simulink model "Ydq_noise_model"  (R2021b)
settings: Solver=FixedStepAuto  StartTime=0.0  StopTime=t_end  FixedStep=1e-5  RelTol=1e-3
undefined symbols (not defined in the file or in its folder): base, omega0, V0, V_p
libraries: spsControlledVoltageSourceLib x3, simulink x2, spsGroundLib x2, spsabctodq0Lib x1, spsdq0toabcLib x1, spsThreePhaseVIMeasurementLib x1, spspowerguiLib x1
settings Model: Creator=lpwoolcock  LastModifiedBy=lpwoolcock
settings SolverCC: AlgebraicLoopSolver=TrustRegion
settings DebuggingCC: SFMachineParentedDataDiag=warning

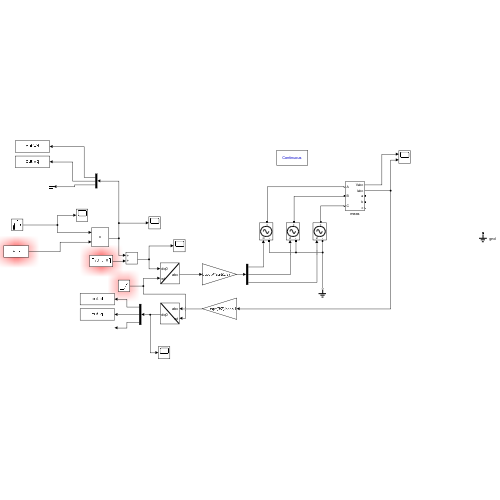
[thumbnail: Simulink's stored preview of the top-level diagram]
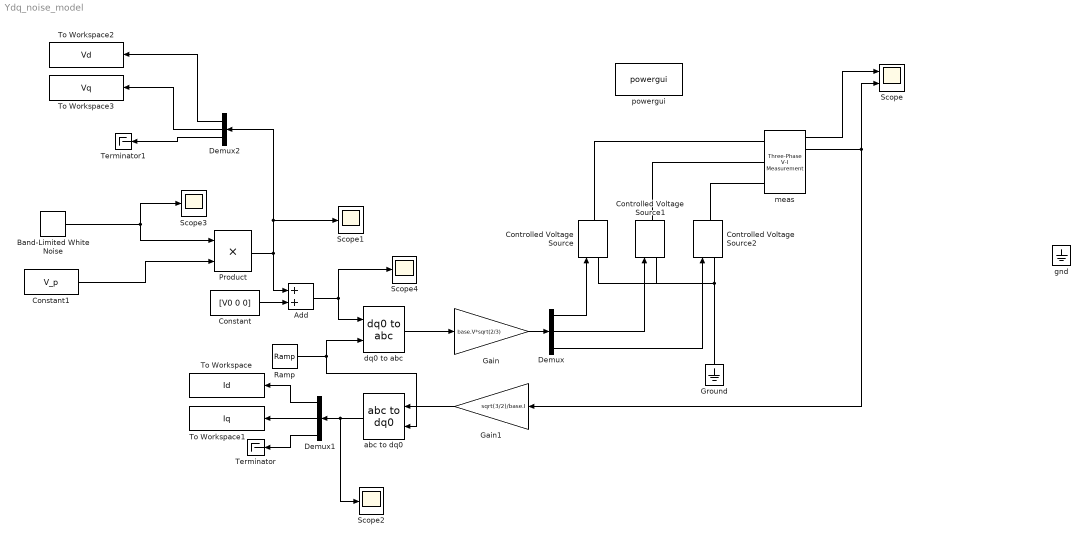
== system Ydq_noise_model ==
  Add : Sum
  Band-Limited White Noise : simulink/Sources/Band-Limited White Noise  Cov=1e-5  Ts=1e-5  seed=[23341]
  Constant : Constant  Value=[V0 0 0]
  Constant1 : Constant  Value=V_p
  Controlled Voltage Source : spsControlledVoltageSourceLib/Controlled Voltage Source  Initialize=off  Source_Type=AC  Amplitude=0  Phase=0  Frequency=0  Measurements=None
  Controlled Voltage Source1 : spsControlledVoltageSourceLib/Controlled Voltage Source  Initialize=off  Source_Type=AC  Amplitude=0  Phase=0  Frequency=0  Measurements=None
  Controlled Voltage Source2 : spsControlledVoltageSourceLib/Controlled Voltage Source  Initialize=off  Source_Type=AC  Amplitude=0  Phase=0  Frequency=0  Measurements=None
  Demux : Demux  Outputs=3
  Demux1 : Demux  Outputs=3
  Demux2 : Demux  Outputs=3
  Gain : Gain  Gain=base.V*sqrt(2/3)
  Gain1 : Gain  Gain=sqrt(3/2)/base.I
  Ground : spsGroundLib/Ground  LConnTagsString=a
  Product : Product
  Ramp : simulink/Sources/Ramp  slope=omega0*base.omega  start=0  InitialOutput=0
  Scope : Scope  NumInputPorts=2
  Scope{1..4} (4 alike) : Scope
  Terminator : Terminator
  Terminator1 : Terminator
  To Workspace : ToWorkspace  VariableName=Id  SaveFormat=Timeseries  SampleTime=-1
  To Workspace1 : ToWorkspace  VariableName=Iq  SaveFormat=Timeseries  SampleTime=-1
  To Workspace2 : ToWorkspace  VariableName=Vd  SaveFormat=Timeseries  SampleTime=-1
  To Workspace3 : ToWorkspace  VariableName=Vq  SaveFormat=Timeseries  SampleTime=-1
  abc to dq0 : spsabctodq0Lib/abc to dq0  Alignment=90 degrees behind phase A axis
  dq0 to abc : spsdq0toabcLib/dq0 to abc  Alignment=90 degrees behind phase A axis
  gnd : spsGroundLib/Ground  LConnTagsString=a
  meas : spsThreePhaseVIMeasurementLib/Three-Phase V-I Measurement  VoltageMeasurement=phase-to-ground  SetLabelV=off  LabelV=Vabc  Vpu=off  VpuLL=off  CurrentMeasurement=yes  SetLabelI=off  LabelI=Iabc  Ipu=off  Pbase=100e6  Vbase=500e3  OutputType=Complex  PhasorSimulation=off  PSBequivalent=0
  powergui : spspowerguiLib/powergui  Priority=1  SimulationMode=Continuous  SampleTime=50e-6  frequency=60  Iterations=50  frequencyindice=0  Pbase=100e6  ErrMax=1e-4  UnitsV=kV  UnitsW=MW  buscounter=0  FunctionMessages=off  echomessages=off  EnableUseOfTLC=off  CurrentSourceSwitches=off  DisableSnubberDevices=off  DisableRonSwitches=off  DisableVfSwitches=off  DisplayEquations=off  AutomaticDiscreteSolvers=off  SolverType=Tustin/Backward Euler (TBE)  Interpol=off  ExternalGateDelay=off  methode=off  Ts=100  x0status=blocks  SPID=on  SwTol=0  HookPort=off  NonlinearTolerance=1e-4  nMaxIteration=100  ContinueOnMaxIteration=off  RestoreLinks=warning  ResistiveCurrentMeasurement=off  Frange=[0:2:500]  Ylog=off  Xlog=on  ShowGrid=off  save=off  variable=ZData  structure=0  ZoomFFT=off  StartTime=0.0  cycles=1  DisplayStyle=1  fundamental=60  FreqAxis=off  MaxFrequency=1000  frequencyindicesteady=1  RmsSteady=1  display=off
  wires:
  Demux/1 -> Controlled Voltage Source/1
  Demux/2 -> Controlled Voltage Source1/1
  Demux/3 -> Controlled Voltage Source2/1
  Ramp/1 -> abc to dq0/2, dq0 to abc/2
  dq0 to abc/1 -> Gain/1
  Gain/1 -> Demux/1
  meas/1 -> Scope/1
  meas/2 -> Gain1/1, Scope/2
  Gain1/1 -> abc to dq0/1
  abc to dq0/1 -> Scope2/1, Demux1/1
  Demux1/1 -> To Workspace/1
  Demux1/2 -> To Workspace1/1
  Demux1/3 -> Terminator/1
  Constant/1 -> Add/2
  Add/1 -> dq0 to abc/1, Scope4/1
  Constant1/1 -> Product/2
  Band-Limited White Noise/1 -> Scope3/1, Product/1
  Demux2/3 -> Terminator1/1
  Demux2/2 -> To Workspace3/1
  Demux2/1 -> To Workspace2/1
  Product/1 -> Demux2/1, Scope1/1, Add/1
  connections:
  Ground/LConn1 -- Controlled Voltage Source/LConn1 -- Controlled Voltage Source1/LConn1 -- Controlled Voltage Source2/LConn1
  meas/LConn1 -- Controlled Voltage Source/RConn1
  meas/LConn2 -- Controlled Voltage Source1/RConn1
  meas/LConn3 -- Controlled Voltage Source2/RConn1
